simulink model "budynek"  (R2013a)
settings: Solver=ode4  StartTime=0.0  StopTime=86400  FixedStep=1  RelTol=1e-3
values from neighbouring files (symbols this model uses):
  cb = 1000    [runme.m]
  ch = 2700    [runme.m]
  cw = 4200    [runme.m]
  dzeta = 1000    [runme.m]
  Fcob = 40    [runme.m]
  Kd = 50    [runme.m]
  kext = 15000    [runme.m]
  kh = 12000    [runme.m]
  Ki = 0.0005    [runme.m]
  Kp = 0.5    [runme.m]
  mb = 20000    [runme.m]
  mh = 3000    [runme.m]
  SP = 20    [runme.m]
  To = 0    [runme.m]
  Tpco0 = 0    [runme.m]
  Tr0 = 0    [runme.m]
  Tzco = 70    [runme.m]
settings Model: Creator=michal  LastModifiedBy=michal
settings DataIOCC: LimitDataPoints=off  SaveOutput=off

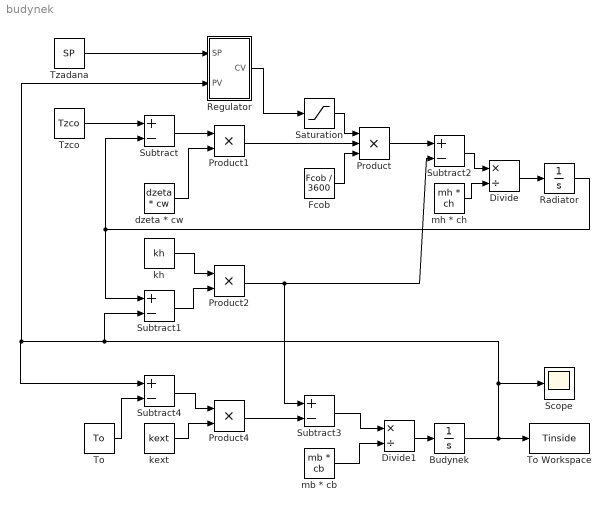
== system budynek ==
  Budynek : Integrator  InitialCondition=Tr0
  Divide : Product  Inputs=*/
  Divide1 : Product  Inputs=*/
  Fcob : Constant  Value=Fcob / 3600
  Product : Product  Inputs=3
  Product1 : Product
  Product2 : Product
  Product4 : Product
  Radiator : Integrator  InitialCondition=Tpco0
  Regulator : Subsystem
  Saturation : Saturate  UpperLimit=1  LowerLimit=0
  Scope : Scope
      settings: YMin=0  YMax=30
  Subtract{,1..4} (5 alike) : Sum  Inputs=+-
  To : Constant  Value=To
  To Workspace : ToWorkspace  VariableName=Tinside  SampleTime=-1
  Tzadana : Constant  Value=SP
  Tzco : Constant  Value=Tzco
  dzeta * cw : Constant  Value=dzeta * cw
  kext : Constant  Value=kext
  kh : Constant  Value=kh
  mb * cb : Constant  Value=mb * cb
  mh * ch : Constant  Value=mh * ch
  wires:
  Tzadana/1 -> Regulator/1(SP)
  Saturation/1 -> Product/1
  Tzco/1 -> Subtract/1
  Radiator/1 -> Subtract1/1, Subtract/2
  Subtract/1 -> Product1/1
  Product1/1 -> Product/2
  dzeta * cw/1 -> Product1/2
  Subtract1/1 -> Product2/2
  Product/1 -> Subtract2/1
  Product2/1 -> Subtract3/1, Subtract2/2
  Subtract2/1 -> Divide/1
  mh * ch/1 -> Divide/2
  Divide/1 -> Radiator/1
  Divide1/1 -> Budynek/1
  mb * cb/1 -> Divide1/2
  Subtract3/1 -> Divide1/1
  Product4/1 -> Subtract3/2
  kh/1 -> Product2/1
  Subtract4/1 -> Product4/1
  kext/1 -> Product4/2
  To/1 -> Subtract4/2
  Budynek/1 -> To Workspace/1, Regulator/2(PV), Subtract4/1, Subtract1/2, Scope/1
  Fcob/1 -> Product/3
  Regulator/1(CV) -> Saturation/1

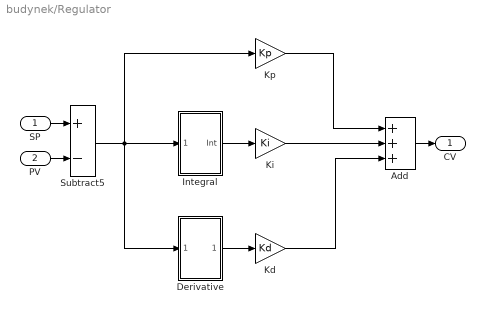
== system budynek/Regulator ==
  SP : Inport
  PV : Inport  Port=2
  Add : Sum  Inputs=+++
  Derivative : Subsystem
  Integral : Subsystem
  Kd : Gain  Gain=Kd
  Ki : Gain  Gain=Ki
  Kp : Gain  Gain=Kp
  Subtract5 : Sum  Inputs=+-
  CV : Outport
  wires:
  Add/1 -> CV/1
  SP/1 -> Subtract5/1
  Kp/1 -> Add/1
  Subtract5/1 -> Derivative/1(Error), Integral/1(Error), Kp/1
  PV/1 -> Subtract5/2
  Integral/1(Int) -> Ki/1
  Ki/1 -> Add/2
  Derivative/1(Der) -> Kd/1
  Kd/1 -> Add/3

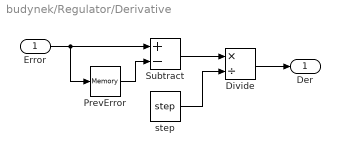
== system budynek/Regulator/Derivative ==
  Error : Inport
  Divide : Product  Inputs=*/
  PrevError : Memory
  Subtract : Sum  Inputs=+-
  step : Constant  Value=step
  Der : Outport
  wires:
  Error/1 -> Subtract/1, PrevError/1
  PrevError/1 -> Subtract/2
  Subtract/1 -> Divide/1
  step/1 -> Divide/2
  Divide/1 -> Der/1

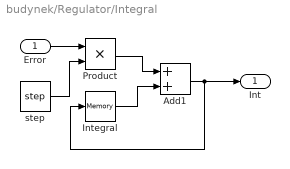
== system budynek/Regulator/Integral ==
  Error : Inport
  Add1 : Sum
  Integral : Memory
  Product : Product
  step : Constant  Value=step
  Int : Outport
  wires:
  Integral/1 -> Add1/2
  step/1 -> Product/2
  Product/1 -> Add1/1
  Error/1 -> Product/1
  Add1/1 -> Int/1, Integral/1
